simulink model "AN_Simulink_Model_v1"  (R2019b)
settings: Solver=VariableStepAuto  StartTime=0.0  StopTime=testtime  RelTol=1e-3
InitFcn:
  | AN_InitFcn_Callback
StopFcn:
  | AN_StopFcn_Callback
values from neighbouring files (symbols this model uses):
  alpha1 = 1.5e-6*100e3    (= 0.15)    [AN_Get_Model_Parameters.m]
  alpha2 = 1e-2*100e3    (= 1000)    [AN_Get_Model_Parameters.m]
  C1initphase = C1initphase + atan(CF/(-rzero))-atan((CF-pimag(2*i-1))/(-preal(2*i-1)))-atan((CF+pimag(2*i-1))/(-preal(2*i-1)))    [AN_Get_Model_Parameters.m]
  c1LPihc = ( Cihc - 2*pi*Fcihc ) / ( Cihc + 2*pi*Fcihc )    [AN_Get_Model_Parameters.m]
  c1LPohc = ( Cohc - 2*pi*Fcohc ) / ( Cohc + 2*pi*Fcohc )    [AN_Get_Model_Parameters.m]
  C1slope = 0.1    [AN_Get_Model_Parameters.m]
  c2LPihc = 2*pi*Fcihc / (2*pi*Fcihc + Cihc)    [AN_Get_Model_Parameters.m]
  c2LPohc = 2*pi*Fcohc / (2*pi*Fcohc + Cohc)    [AN_Get_Model_Parameters.m]
  C2slope = 0.2    [AN_Get_Model_Parameters.m]
  centerfreq = 165.4*(10^((bmplace+1.2)/(35/2.1)) - 1.0)    [AN_Get_Model_Parameters.m]
  CF = 2*pi*cf    [AN_Get_Model_Parameters.m]
  cf_factor = min(cfsat, 10^(cfslope*cf/1e3 + cfconst)) * 2.0    [AN_Get_Model_Parameters.m]
  cordiciterationswb = 52    [AN_Get_Model_Parameters.m]
  delta_phase = -2*pi*centerfreq*tdres    [AN_Get_Model_Parameters.m]
  fs_bilinear = 2*pi*cf/tan(2*pi*cf*tdres/2)    [AN_Get_Model_Parameters.m]
  gainihc = 1.0    (= 1)    [AN_Get_Model_Parameters.m]
  gainohc = 1.0    (= 1)    [AN_Get_Model_Parameters.m]
  ihcasym = 3.0    (= 3)    [AN_Get_Model_Parameters.m]
  m11 = 1/(C^2+5.9761e+003*C+2.5255e+007)    [AN_Get_Model_Parameters.m]
  m12 = -2*C^2+2*2.5255e+007    [AN_Get_Model_Parameters.m]
  m13 = C^2-5.9761e+003*C+2.5255e+007    [AN_Get_Model_Parameters.m]
  m14 = C^2+5.6665e+003*C    [AN_Get_Model_Parameters.m]
  m15 = -2*C^2    [AN_Get_Model_Parameters.m]
  m16 = C^2-5.6665e+003*C    [AN_Get_Model_Parameters.m]
  m21 = 1/(C^2+6.4255e+003*C+1.3975e+008)    [AN_Get_Model_Parameters.m]
  m22 = -2*C^2+2*1.3975e+008    [AN_Get_Model_Parameters.m]
  m23 = C^2-6.4255e+003*C+1.3975e+008    [AN_Get_Model_Parameters.m]
  m24 = C^2+5.8934e+003*C+1.7926e+008    [AN_Get_Model_Parameters.m]
  m25 = -2*C^2+2*1.7926e+008    [AN_Get_Model_Parameters.m]
  m26 = C^2-5.8934e+003*C+1.7926e+008    [AN_Get_Model_Parameters.m]
  m31 = 1/(C^2+2.4891e+004*C+1.2700e+009)    [AN_Get_Model_Parameters.m]
  m32 = -2*C^2+2*1.2700e+009    [AN_Get_Model_Parameters.m]
  m33 = C^2-2.4891e+004*C+1.2700e+009    [AN_Get_Model_Parameters.m]
  m34 = (3.1137e+003*C+6.9768e+008)    [AN_Get_Model_Parameters.m]
  m35 = 2*6.9768e+008    (= 1395360000)    [AN_Get_Model_Parameters.m]
  m36 = -3.1137e+003*C+6.9768e+008    [AN_Get_Model_Parameters.m]
  megainmax = 2    [AN_Get_Model_Parameters.m]
  minR = 0.05    [AN_Get_Model_Parameters.m]
  multFac = max(2.95*max(1.0,1.5-spont/100), 4.3-0.2*cf/1e3)    [AN_Get_Model_Parameters.m]
  norm_gainc1 = single(norm_gainc1)    [AN_Get_Model_Parameters.m]
  nSites = single(4)    [AN_Get_Model_Parameters.m]
  ohcasym = 7.0    (= 7)    [AN_Get_Model_Parameters.m]
  order_of_zero = half_order_pole    (= 5)    [AN_Get_Model_Parameters.m]
  pimag = zeros(11,1)    [AN_Get_Model_Parameters.m]
  preal = zeros(11,1)    [AN_Get_Model_Parameters.m]
  s0 = 12.0    (= 12)    [AN_Get_Model_Parameters.m]
  s1 = 5.0    (= 5)    [AN_Get_Model_Parameters.m]
  shift = 1.0/(1.0+ohcasym)    (= 0.125)    [AN_Get_Model_Parameters.m]
  spont = 100    [AN_Get_Model_Parameters.m]
  strength = (20.0e6)/(10^(corner/20))    (= 2000)    [AN_Get_Model_Parameters.m]
  tauwb = TauWBMax + (bmTaubm-bmTaumax)*(TauWBMax-TauWBMin)/(bmTaumax-bmTaumin)    [AN_Get_Model_Parameters.m]
  TauWBMax = Taumin + 0.2*(Taumax-Taumin)    [AN_Get_Model_Parameters.m]
  TauWBMin = TauWBMax/Taumax*Taumin    [AN_Get_Model_Parameters.m]
  wborder = 3    [AN_Get_Model_Parameters.m]
  x0 = s0*log((1.0/shift-1)/(1+exp(x1/s1)))    [AN_Get_Model_Parameters.m]
  x1 = 5.0    (= 5)    [AN_Get_Model_Parameters.m]
undefined symbols (not defined in the file or in its folder): bmTaumax, bmTaumin, cf, cihc, cohc, dfilt, Fs, jsin, norm_gainc2, tabs, tdres, trel, wbgain
libraries: dsparch4 x7, simulink x6, dspsrcs4 x3
(part 1 of 2)
settings Model: NumberOfSteps=50  Creator=mblun  LastModifiedBy=t96f346
settings OptimizationCC: BlockReduction=off  ConditionallyExecuteInputs=off  DefaultParameterBehavior=Inlined
settings DebuggingCC: UnderSpecifiedDimensionMsg=warning
settings SFSimCC: CustomCodeUndefinedFunction=UseInterfaceOnly

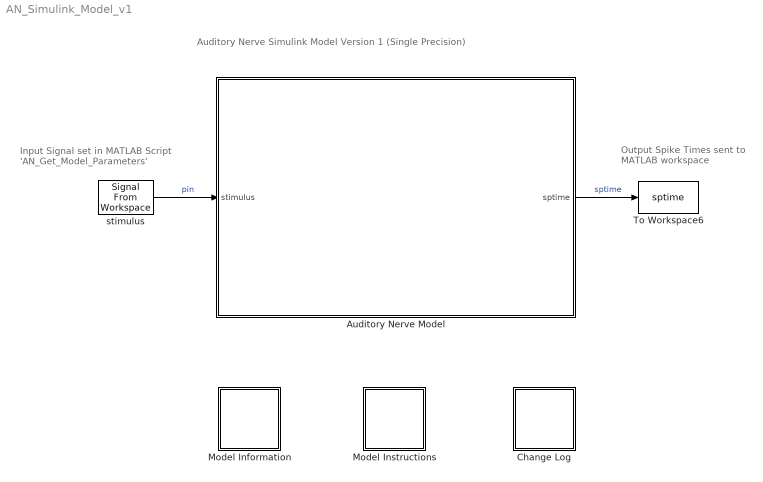
== system AN_Simulink_Model_v1 ==
  note: Input Signal set in MATLAB Script 'AN_Get_Model_Parameters'
  note: Auditory Nerve Simulink Model Version 1 (Single Precision)
  note: Output Spike Times sent to MATLAB workspace
  Auditory Nerve Model : Subsystem
  Change Log : Subsystem
  Model Information : Subsystem
  Model Instructions : Subsystem
  To Workspace6 : ToWorkspace  VariableName=sptime  SampleTime=-1
      settings: Save2DSignal=2-D array (concatenate along first dimension)
  "stimulus " : dspsrcs4/Signal From Workspace  X=RxSignal  Ts=tdres  nsamps=1  OutputAfterFinalValue=Setting to zero  ignoreOrWarnInputAndFrameLengths=off  OutputFrames=off
  wires:
  Auditory Nerve Model/1(sptime) -> To Workspace6/1  "sptime"
  "stimulus "/1 -> Auditory Nerve Model/1(stimulus)  "pin"

== system AN_Simulink_Model_v1/Auditory Nerve Model ==
  note: IHC
  note: OHC
  note: Input sound pressure waveform passes through middle ear filter
  note: Middle Ear output signal goes through broadly-tuned C2 filter and narrowly-tuned C1 filter in the model signal path
  note: C1/C2-filtered signals pass through the inner hair cell model (IHC), resulting in a relative transmembrane potential output
  note: Relative potential from IHC passes through the synapse model, which outputs the mean synaptic release rate of the neuron
  note: Mean synaptic release rate is input to the spike generator model, which uses a pseudo-random process to determine spike times for the neuron, along with various firing statistics of the neuron
  note: Middle Ear output signal goes through the gammatone filter of the control path. This is a feed-forward path which is used to tune the highly-sensitive C1 filter
  note: Gammatone filter output is passed to the outer-hearing cell model (OHC), which outputs a time constant to be used by the C1 filter
  note: The C1 filter time constant is input to a function which feeds an updated time-constant and associated gain back into the gammatone control path filter
  stimulus : Inport
  C1 Chirp Filter : Subsystem
  C2 Wideband Filter : Subsystem
  CP Wideband Gammatone Filter : Subsystem
  Middle Ear Filter : Subsystem
  Spike Generator : Subsystem
  Subsystem : Subsystem
  Subsystem1 : Subsystem
  Synapse Model : Subsystem
  f(tauc1) : Subsystem
  sptime : Outport  VectorParamsAs1DForOutWhenUnconnected=off
  wires:
  CP Wideband Gammatone Filter/1(output1) -> Subsystem1/1(wbout)  "wbout1"
  f(tauc1)/1(tauwb) -> CP Wideband Gammatone Filter/2(tauwb)  "tauwb"
  Subsystem1/1(tauc1) -> f(tauc1)/1(tauc1), C1 Chirp Filter/2(tauc1)  "tauc1"
  Middle Ear Filter/1(output) -> CP Wideband Gammatone Filter/3(stimulus), C1 Chirp Filter/1(meout), C2 Wideband Filter/1(stimulus)  "meout"
  stimulus/1 -> Middle Ear Filter/1(stimulus)  "pin"
  C1 Chirp Filter/1(output) -> Subsystem/2(C1filterout)  "C1filterout"
  Subsystem/1(ihcout) -> Synapse Model/1(ihcout)  "ihcout"
  C2 Wideband Filter/1(output) -> Subsystem/1(C2filterout)  "C2filterout"
  f(tauc1)/2(wbgain) -> CP Wideband Gammatone Filter/1(wbgain)  "wbgain"
  Synapse Model/1(synout) -> Spike Generator/1(synout)  "synout"
  Spike Generator/1(sptime) -> sptime/1  "sptime"

== system AN_Simulink_Model_v1/Change Log ==
  Change Log : simulink/Model-Wide Utilities/Model Info  Frame=on  DisplayStringWithTags=|  HorizontalTextAlignment=Left  LeftAlignmentValue=0.02
      | The following is the change log for the AN Simulink Model. Any major version changes should be 
      | documented and summarized below.
      | 
      | ------------------------------------------------------------------------------------------------------------------------------------
      | 
      | Version 1:
      | 	
      | 	- First Draft Version of Simulink Model by Matthew Blunt --- 08/07/2019
      | 
      | ------------------------------------------------------------------------------------------------------------------------------------
      | 
      | (Next Version Here)
      | 
      | 	- (Details and Changes Here)

== system AN_Simulink_Model_v1/Model Information ==
  "Model Information " : simulink/Model-Wide Utilities/Model Info  Frame=on  DisplayStringWithTags=|  HorizontalTextAlignment=Left  LeftAlignmentValue=0.02
      | Model Name: AN_Simulink_Model_v1
      | Created By: Matthew Blunt
      | Last Modification Date: 08/07/2019
      | Most Recently Modified By: Matthew Blunt
      | Model Version: 1
      | 
      | ------------------------------------------------------------------------------------------------------------------------------------
      | 
      | Description: This is a sample-based auditory nerve Simulink model, designed to closely replicate the 
      | auditory nerve model presented in the following publication:
      | 
      | 			Bruce, I.C., Erfani, Y., and Zilany, M.S.A. (2018). "A Phenomenological
      | 			model of the synapse between the inner hair cell and auditory nerve: 
      | 			Implications of limited neurotransmitter release sites," to appear in
      | 			Hearing Research. (Special Issue on "Computational Models in Hearing".)
      | 
      | It is important to also recognize the previous iterations of the phenomenological auditory 
      | nerve model, as they served as additional references during the design of the Simulink model.
      | 
      | ------------------------------------------------------------------------------------------------------------------------------------
      | 
      | This software was developed in conjunction with Flat Earth Inc
      | 
      | Copyright 2019 Flat Earth Inc
      | 
      | THE SOFTWARE IS PROVIDED "AS IS", WITHOUT WARRANTY OF ANY KIND, EXPRESS OR
      | IMPLIED, INCLUDING BUT NOT LIMITED TO THE WARRANTIES OF MERCHANTABILITY,
      | FITNESS FOR A PARTICULAR PURPOSE AND NONINFRINGEMENT. IN NO EVENT SHALL
      | THE AUTHORS OR COPYRIGHT HOLDERS BE LIABLE FOR ANY CLAIM, DAMAGES OR
      | OTHER LIABILITY, WHETHER IN AN ACTION OF CONTRACT, TORT OR OTHERWISE,
      | ARISING FROM, OUT OF OR IN CONNECTION WITH THE SOFTWARE OR THE USE OR
      | OTHER DEALINGS IN THE SOFTWARE.
      | 
      |    		Matthew Blunt
      |   		 Flat Earth Inc
      |    		985 Technology Blvd
      |    		Bozeman, MT 59718
      |    		support@flatearthinc.com

== system AN_Simulink_Model_v1/Model Instructions ==
  "Model Instructions " : simulink/Model-Wide Utilities/Model Info  Frame=on  DisplayStringWithTags=|  HorizontalTextAlignment=Left  LeftAlignmentValue=0.02
      | The following is a full set of instructions outlining the necessary steps to be taken in order to run the 
      | AN Simulink Model. Instructions can also be found in the readme file found in the
      | AN_Simulink_Model_v1_Doubles folder.
      | 
      | ------------------------------------------------------------------------------------------------------------------------------------
      | 
      | ** Quick Start Instructions **
      | 
      | If the user desires to simply run the model as is, refer to the Quick Start
      | Instructions pdf, which gives a quick visual tutorial on running the Auditory
      | Nerve Simulink Model.
      | 
      | ------------------------------------------------------------------------------------------------------------------------------------
      | 
      | ** Modify Model Instructions **
      | 
      | If the user desires to make modifications to the model before runtime,
      | refer to the Modify Model Instructions pdf, which gives a quick visual
      | tutorial on modifying the Auditory Nerve Simulink Model.
      | 
      | ------------------------------------------------------------------------------------------------------------------------------------
      | 
      | ** Verify Model Instructions **
      | 
      | If the user desires to verify model functionality against the original 
      | model source code, instructions are listed below, as well as in the readme.txt file
      | 
      | 1. Make sure MATLAB R2019a and a compatible C compiler are downloaded on the
      | machine the model will be running on. The C compiler is needed for C functions
      | used in the test/verification process. The compiler used for testing was the
      | MinGW-w64 C/C++ Compiler. This can be easily accessed for free in the Add-On
      | Explorer found in the MATLAB home tab.
      | 
      | 2. Open the AN_Simulink_Model_v1_Doubles folder in MATLAB. This is necessary in
      | order for the Simulink model to interact with MATLAB.
      | 
      | 3. Edit model parameters, if necessary. This can be done by adjusting the
      | overall model parameters set in the AN_Set_Model_Parameters script, or adjusting
      | other parameters in the AN_Get_Model_Parameters script. Both scripts are found
      | in the AN_Simulink_Model_v1_Doubles folder.
      | 
      | 4. Set the 'verificationflag' boolean to 'true' in the AN_Set_Model_Parameters
      | script. This enables the model to run the comparison C/MATLAB source functions
      | which are compared to the Simulink Model.
      | 
      | 5. Run the model. This is done by simply clicking the green 'Run' button
      | located at the top panel of Simulink. In addition, the model can be stepped
      | through in increments, using the 'Step Through' button to the right of the
      | 'Run' button.

== system AN_Simulink_Model_v1/Auditory Nerve Model/C1 Chirp Filter ==
  note: C1 Chirp Filter:
      |
      | Inputs : ME Filtered Signal (meout)
      | C1 Coefficients (a&b)
      | Normalizing Gain (norm_gain)
      |
      | Output : C1 Filtered Signal (c1filterout)
      |
      | - 10th Order IIR Bandpass Filter
      |
      | - Coefficients are determined in previous Get C1 Coefficients block
      |
      | - Implemented w/ Simulink biquad block
  note: Get C1 Coefficients
      |
      | Input : Pole-Shifting Feedback Parameter (rsigma)
      |
      | Outputs : C1 Coefficients (a&b)
      | Normalizing Gain (norm_gain)
      |
      | - Consists of various calculations to shift continuous-time pole locations according to rsigma feedback, then apply a bilinear transformation to bring the poles to the digital space before finding the coefficients for the C1 filter
  note: Calculate C1 Filter Output
      |
      | - Simply scale the output by cihc
  note: Calculate Pole-Shifting Parameter rsigma
      |
      | Input : C1 Feedback Time Constant (tauc1)
      |
      | Outputs : Pole-Shifting Parameter rsigma
      |
      | - Simple calculation to find rsigma from time constant feedback input
  meout : Inport
  tauc1 : Inport  Port=2
  C1 FIlter : Subsystem
  Calculate C1filterout : Subsystem
  Calculate rsigma : Subsystem
  Get C1 Coefficients : Subsystem
  To Workspace2 : ToWorkspace  VariableName=rsigma  SampleTime=-1
      settings: Save2DSignal=2-D array (concatenate along first dimension)
  output : Outport  VectorParamsAs1DForOutWhenUnconnected=off
  wires:
  meout/1 -> C1 FIlter/1(meout)
  C1 FIlter/1(Out1) -> Calculate C1filterout/1(C1filterouttmp)  "c1filterouttmp"
  Get C1 Coefficients/1(b0(5)) -> C1 FIlter/2(b0(5))
  Get C1 Coefficients/2(b0(3)) -> C1 FIlter/3(b0(3))
  Get C1 Coefficients/3(b0(1)) -> C1 FIlter/4(b0(1))
  Get C1 Coefficients/4(b1(5)) -> C1 FIlter/5(b1(5))
  Get C1 Coefficients/5(b1(3)) -> C1 FIlter/6(b1(3))
  Get C1 Coefficients/6(b1(1)) -> C1 FIlter/7(b1(1))
  Get C1 Coefficients/7(b2(5)) -> C1 FIlter/8(b2(5))
  Get C1 Coefficients/8(b2(3)) -> C1 FIlter/9(b2(3))
  Get C1 Coefficients/9(b2(1)) -> C1 FIlter/10(b2(1))
  Get C1 Coefficients/10(a2(5)) -> C1 FIlter/11(a2(5))
  Get C1 Coefficients/11(a2(3)) -> C1 FIlter/12(a2(3))
  Get C1 Coefficients/12(a2(1)) -> C1 FIlter/13(a2(1))
  Get C1 Coefficients/13(a1(1)) -> C1 FIlter/14(a1(1))
  Get C1 Coefficients/14(a1(3)) -> C1 FIlter/15(a1(3))
  Get C1 Coefficients/15(a1(5)) -> C1 FIlter/16(a1(5))
  Calculate C1filterout/1(C1filterout) -> output/1  "C1filterout"
  Calculate rsigma/1(rsigma) -> Get C1 Coefficients/1(rsigma), To Workspace2/1  "rsigma"
  tauc1/1 -> Calculate rsigma/1(tauc1)  "tauc1"

== system AN_Simulink_Model_v1/Auditory Nerve Model/C2 Wideband Filter ==
  note: C2 Wideband Filter:
      |
      | Input : ME Filtered Signal (meout)
      |
      | Output : C2 Filtered Signal (c2filterout)
      |
      | - 10th Order IIR Bandpass Filter
      |
      | - Coefficients are determined in AN_Get_Parameters init script
      |
      | - Implemented w/ Simulink biquad block
  note: Calculate C2 Filter Output:
      |
      | - Simply scale filter output
  stimulus : Inport
  Biquad Filter1 : dsparch4/Biquad Filter  FilterSource=Dialog parameters  CoeffSource=Specify via dialog  FilterObject=dfilt.df2tsos([1 0.3 0.4],[1 0.1 0.2])  IIRFiltStruct=Direct form II transposed  BiQuadCoeffs=C2coeffs  ScaleValues=1  IC=0  ICnum=0  ICden=0  a0Flag=Warning  optimizeScaleValues=on  ScaleValueMode=Specify via input port (g)  roundingMode=Floor  overflowMode=on  scaleValueFracLength=14  denProdOutputFracLength=30  denAccumFracLength=30  secondMemoryFracLength=15
      settings: SourceProductName=DSP System Toolbox
  Calculate C2filterout : Subsystem
  Gain : Gain  Gain=norm_gainc2/4
  output : Outport  VectorParamsAs1DForOutWhenUnconnected=off
  wires:
  stimulus/1 -> Biquad Filter1/1
  Biquad Filter1/1 -> Gain/1
  Gain/1 -> Calculate C2filterout/1(C2filterouttmp)  "c2filterouttmp"
  Calculate C2filterout/1(C2filterout) -> output/1  "C2filterout"

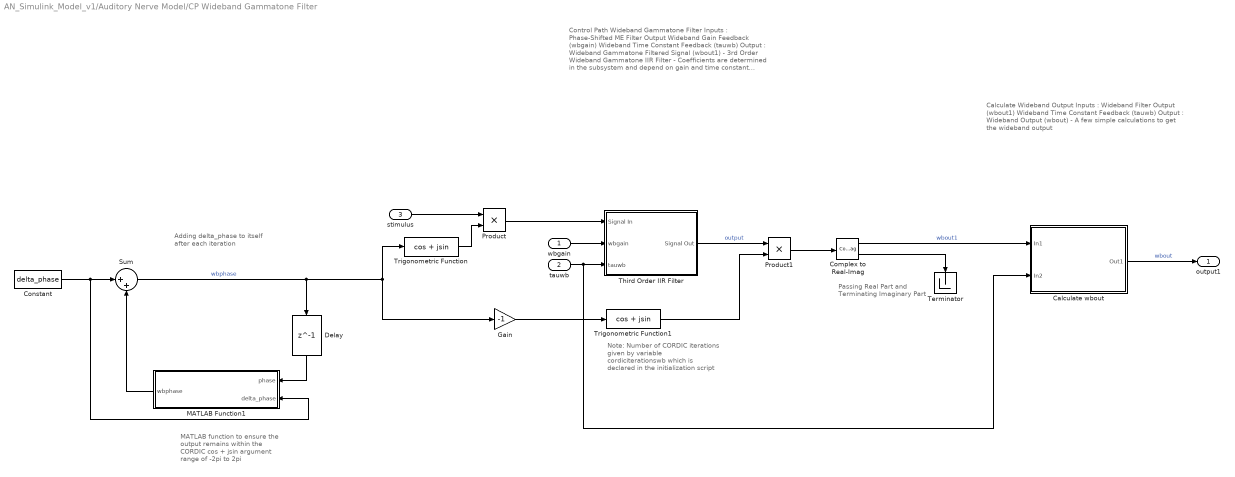
== system AN_Simulink_Model_v1/Auditory Nerve Model/CP Wideband Gammatone Filter ==
  note: Passing Real Part and Terminating Imaginary Part
  note: Note: Number of CORDIC iterations given by variable cordiciterationswb which is declared in the initialization script
  note: Adding delta_phase to itself after each iteration
  note: MATLAB function to ensure the output remains within the CORDIC cos + jsin argument range of -2pi to 2pi
  note: Control Path Wideband Gammatone Filter
      |
      | Inputs : Phase-Shifted ME Filter Output
      | Wideband Gain Feedback (wbgain)
      | Wideband Time Constant Feedback (tauwb)
      |
      | Output : Wideband Gammatone Filtered Signal (wbout1)
      |
      | - 3rd Order Wideband Gammatone IIR Filter
      |
      | - Coefficients are determined in the subsystem and depend on gain and time constant feedback
      |
      | - Implemented w/ Direct Form I Block Structure
  note: Calculate Wideband Output
      |
      | Inputs : Wideband Filter Output (wbout1)
      | Wideband Time Constant Feedback (tauwb)
      |
      | Output : Wideband Output (wbout)
      |
      | - A few simple calculations to get the wideband output
  wbgain : Inport
  tauwb : Inport  Port=2  OutDataTypeStr=single
  stimulus : Inport  Port=3  OutDataTypeStr=single
  Calculate wbout : Subsystem
  Complex to Real-Imag : ComplexToRealImag
  Constant : Constant  Value=delta_phase  OutDataTypeStr=single  SampleTime=-1
  Delay : Delay  DelayLength=1  InitialCondition=0  UseCircularBuffer=on
  Gain : Gain  Gain=-1  OutDataTypeStr=single
  MATLAB Function1 : MATLAB Function  TreatAsAtomicUnit=on
  Product : Product  OutDataTypeStr=single
  Product1 : Product  OutDataTypeStr=single
  Sum : Sum  Inputs=|++  OutDataTypeStr=single
  Terminator : Terminator
  Third Order IIR Filter : Subsystem
  Trigonometric Function : Trigonometry  Operator=cos + jsin  ApproximationMethod=CORDIC  NumberOfIterations=cordiciterationswb
  Trigonometric Function1 : Trigonometry  Operator=cos + jsin  ApproximationMethod=CORDIC  NumberOfIterations=cordiciterationswb
  output1 : Outport  VectorParamsAs1DForOutWhenUnconnected=off
  wires:
  Third Order IIR Filter/1(Signal Out) -> Product1/1  "output"
  Trigonometric Function/1 -> Product/2
  Constant/1 -> Sum/1, MATLAB Function1/2(delta_phase)
  stimulus/1 -> Product/1
  Product/1 -> Third Order IIR Filter/1(Signal In)
  Sum/1 -> Gain/1, Trigonometric Function/1, Delay/1  "wbphase"
  Product1/1 -> Complex to Real-Imag/1
  Complex to Real-Imag/1 -> Calculate wbout/1(In1)  "wbout1"
  Complex to Real-Imag/2 -> Terminator/1
  Gain/1 -> Trigonometric Function1/1
  Trigonometric Function1/1 -> Product1/2
  tauwb/1 -> Calculate wbout/2(In2), Third Order IIR Filter/3(tauwb)
  wbgain/1 -> Third Order IIR Filter/2(wbgain)
  Calculate wbout/1(Out1) -> output1/1  "wbout"
  Delay/1 -> MATLAB Function1/1(phase)
  MATLAB Function1/1(wbphase) -> Sum/2

== system AN_Simulink_Model_v1/Auditory Nerve Model/Middle Ear Filter ==
  note: Middle Ear Filter
      |
      | Input : Pressure Stimulus Waveform (pin or px)
      |
      | Output : Filtered Signal (meout)
      |
      | - 6th Order IIR Lowpass Filter
      |
      | - Coefficients are determined in AN_Get_Parameters init script
      |
      | - Implemented w/ Simulink biquad block
  stimulus : Inport
  Biquad Filter4 : dsparch4/Biquad Filter  FilterSource=Dialog parameters  CoeffSource=Specify via dialog  FilterObject=dfilt.df2tsos([1 0.3 0.4],[1 0.1 0.2])  IIRFiltStruct=Direct form II transposed  BiQuadCoeffs=[m14*m11 m15*m11 m16*m11 1 m12*m11 m13*m11; m24*m21 m25*m21 m26*m21 1 m22*m21 m23*m21; m34*m31 m35*m31 m36*m31 1 m32*m31 m33*m31]  ScaleValues=[1 1 1 1/megainmax]  IC=0  ICnum=0  ICden=0  a0Flag=Warning  optimizeScaleValues=on  ScaleValueMode=Specify via input port (g)  roundingMode=Floor  overflowMode=on  scaleValueFracLength=14  denProdOutputFracLength=30  denAccumFracLength=30  secondMemoryFracLength=15
      settings: SourceProductName=DSP System Toolbox
  To Workspace3 : ToWorkspace  VariableName=meout  SampleTime=-1
      settings: Save2DSignal=2-D array (concatenate along first dimension)
  output : Outport  VectorParamsAs1DForOutWhenUnconnected=off
  wires:
  stimulus/1 -> Biquad Filter4/1
  Biquad Filter4/1 -> To Workspace3/1, output/1  "output"

== system AN_Simulink_Model_v1/Auditory Nerve Model/Spike Generator ==
  note: 4-Site Synaptic Release & Adaptive Redocking
      |
      | Input : Synapse Output (synout) & Uniformly Distributed Random Number Vector between 0 and 1 (randNums)
      |
      | Output : Spike Times (sptime), Spike Count (spCount), Current Redocking Period (current_redocking_period), & Redocking Time Vector (trd_vector)
      |
      | - Implemented using Stateflow Chart and embedded MATLAB functions
      |
      | - Shows states of synaptic sites during simulation
  note: Calculation of Mean Spike Rate
      |
      | Input : Synapse Output (synout) & Redocking Time Vector (trd_vector)
      |
      | Output : Mean Spike Rate (meanrate)
      |
      | - Statistical Estimation of Mean Spike Rate to Account for Random Nature of Spike Generation Process
  synout : Inport
  Calculate Mean Spike Rate : Subsystem
  Random Number Generator : dspsrcs4/Signal From Workspace  X=randNums  Ts=1/Fs  nsamps=1  OutputAfterFinalValue=Setting to zero  ignoreOrWarnInputAndFrameLengths=off  OutputFrames=off
  Stateflow Logic Chart : Stateflow chart  BlockKeywords=__PRM__SERIALIZED__DATA__:Stateflow Chart,Stateflow Diagram  TreatAsAtomicUnit=on
  To Workspace1 : ToWorkspace  VariableName=meanrate  SampleTime=-1
      settings: Save2DSignal=2-D array (concatenate along first dimension)
  To Workspace2 : ToWorkspace  VariableName=trd_vector  SampleTime=-1
      settings: Save2DSignal=2-D array (concatenate along first dimension)
  To Workspace6 : ToWorkspace  VariableName=spCount  SampleTime=-1
      settings: Save2DSignal=2-D array (concatenate along first dimension)
  To Workspace7 : ToWorkspace  VariableName=current_redocking_period  SampleTime=-1
      settings: Save2DSignal=2-D array (concatenate along first dimension)
  sptime : Outport  VectorParamsAs1DForOutWhenUnconnected=off
  wires:
  Stateflow Logic Chart/3(current_redocking_period) -> To Workspace7/1
  Stateflow Logic Chart/4(trd_vector) -> Calculate Mean Spike Rate/2(trd_vector), To Workspace2/1  "trd_vector"
  Stateflow Logic Chart/1(sptime) -> sptime/1
  synout/1 -> Stateflow Logic Chart/1(synout), Calculate Mean Spike Rate/1(synout)  "synout"
  Stateflow Logic Chart/2(spCount) -> To Workspace6/1
  Random Number Generator/1 -> Stateflow Logic Chart/2(randNums)
  Calculate Mean Spike Rate/1(meanrate) -> To Workspace1/1  "meanrate"

== system AN_Simulink_Model_v1/Auditory Nerve Model/Subsystem ==
  note: Sum Nonlinear Function Outputs
  note: IHC C2 Nonlinear Logarithmic Transduction Function
      |
      | Input : C2 Filtered Signal (c2filterout)
      |
      | Output : C2 Transduction Function Output (c2vihctmp)
  note: IHC C1 Nonlinear Logarithmic Transduction Function
      |
      | Input : C1 Filtered Signal (c1filterout)
      |
      | Output : C1 Transduction Function Output (c1vihctmp)
  note: IHC Lowpass Filter
      |
      | Input : Sum of C1 and C2 Nonlinear Outputs (ihcnonlinout)
      |
      | Output : IHC Output (ihcout)
      |
      | - 7th Order IIR Lowpass Filter
      |
      | - Implemented using Simulink biquad
  C2filterout : Inport
  C1filterout : Inport  Port=2
  IHC C1 NL Logarithmic Function : Subsystem
  IHC C2 NL Logarithmic Function : Subsystem
  IHC LP Filter : Subsystem
  Sum1 : Sum  Inputs=|++
  To Workspace : ToWorkspace  VariableName=ihcout  SampleTime=-1
      settings: Save2DSignal=2-D array (concatenate along first dimension)
  ihcout : Outport  VectorParamsAs1DForOutWhenUnconnected=off
  wires:
  IHC C2 NL Logarithmic Function/1(output) -> Sum1/1  "c2vihctmp"
  IHC C1 NL Logarithmic Function/1(output) -> Sum1/2  "c1vihctmp"
  C1filterout/1 -> IHC C1 NL Logarithmic Function/1(stimulus)  "c1filterout"
  IHC LP Filter/1(output) -> To Workspace/1, ihcout/1  "ihcout"
  Sum1/1 -> IHC LP Filter/1(stimulus)  "ihcnonlinout"
  C2filterout/1 -> IHC C2 NL Logarithmic Function/1(stimulus)  "c2filterout"

== system AN_Simulink_Model_v1/Auditory Nerve Model/Subsystem1 ==
  note: OHC Lowpass Filter
      |
      | Inputs : OHC Nonlinear Output (ohcnonlinout)
      |
      | Output : LP Filtered OHC Output (ohcout)
      |
      | - 2nd Order IIR Lowpass Filter
      |
      | - Coefficients are determined in the init script
      |
      | - Implemented w/ Simulink biquad
  note: Nonlinear Function After OHC
      |
      | Input : LP Filtered OHC Output (ohcout)
      |
      | Output : Temporary C1 Time Constant (tmptauc1)
      |
      | - Nonlinear Function designed to convert the Lowpass Filter Output to a Time Varying Constant for the C1 Filter
  note: OHC Nonlinear Boltzman Function
      |
      | Input : Wideband Output (wbout)
      |
      | Output : OHC Nonlinear Output (ohcnonlinout)
      |
      | - 2nd Order Boltzman Function
  note: Calculate C1 Time Constant
      |
      | Input : Temporary C1 Time Constant (tmptauc1)
      |
      | Output : C1 Time Constant (tauc1)
      |
      | - A simple calculation to get the final C1 time constant value
  wbout : Inport
  Calculate tauc1 : Subsystem
  NL After OHC Function : Subsystem
  OHC LP Filter : Subsystem
  OHC NL Boltzman Function : Subsystem
  To Workspace1 : ToWorkspace  VariableName=tauc1  SampleTime=-1
      settings: Save2DSignal=2-D array (concatenate along first dimension)
  tauc1 : Outport  VectorParamsAs1DForOutWhenUnconnected=off
  wires:
  wbout/1 -> OHC NL Boltzman Function/1(stimulus)  "wbout"
  NL After OHC Function/1(output) -> Calculate tauc1/1(In1)  "tmptauc1"
  OHC LP Filter/1(output) -> NL After OHC Function/1(stimulus)  "ohcout"
  OHC NL Boltzman Function/1(output) -> OHC LP Filter/1(stimulus)  "ohcnonlinout"
  Calculate tauc1/1(Out1) -> To Workspace1/1, tauc1/1  "tauc1"

== system AN_Simulink_Model_v1/Auditory Nerve Model/Synapse Model ==
  note: NL Before PLA
      |
      | Input : IHC output (ihcout)
      |
      | Output : Power Law Adaptation Input (powerLawIn)
      |
      | - Adapted slightly from source code in order to avoid log10(0)
  ihcout : Inport
  NL Before PLA : Subsystem
  Power Law Adaptation : Subsystem
  synout : Outport  VectorParamsAs1DForOutWhenUnconnected=off
  wires:
  ihcout/1 -> NL Before PLA/1(ihcout)  "ihcout"
  NL Before PLA/1(powerLawIn) -> Power Law Adaptation/1(powerLawIn)  "powerLawIn"
  Power Law Adaptation/1(synout) -> synout/1  "synout"

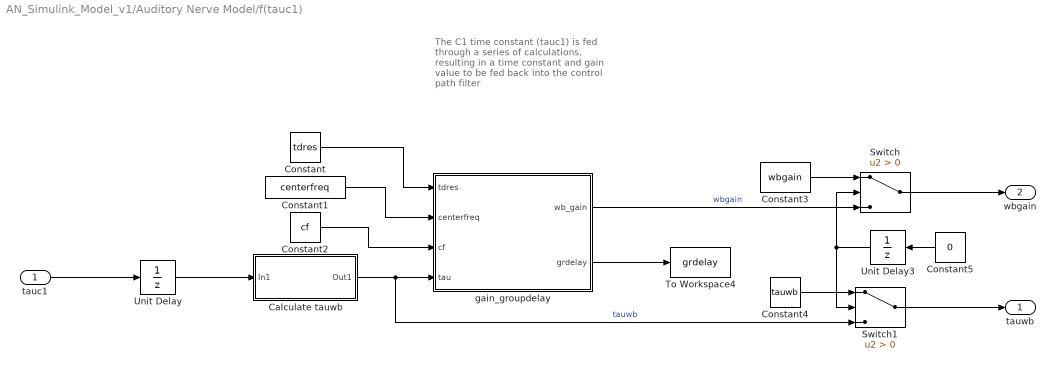
== system AN_Simulink_Model_v1/Auditory Nerve Model/f(tauc1) ==
  note: The C1 time constant (tauc1) is fed through a series of calculations, resulting in a time constant and gain value to be fed back into the control path filter
  tauc1 : Inport
  Calculate tauwb : Subsystem
  Constant : Constant  Value=tdres  OutDataTypeStr=single  SampleTime=-1
  Constant1 : Constant  Value=centerfreq  OutDataTypeStr=single  SampleTime=-1
  Constant2 : Constant  Value=cf  OutDataTypeStr=single  SampleTime=-1
  Constant3 : Constant  Value=wbgain  OutDataTypeStr=single  SampleTime=-1
  Constant4 : Constant  Value=tauwb  OutDataTypeStr=single  SampleTime=-1
  Constant5 : Constant  Value=0  OutDataTypeStr=single  SampleTime=-1
  Switch : Switch  Criteria=u2 > Threshold
  Switch1 : Switch  Criteria=u2 > Threshold
  To Workspace4 : ToWorkspace  VariableName=grdelay  SampleTime=-1
      settings: Save2DSignal=2-D array (concatenate along first dimension)
  Unit Delay : UnitDelay  SampleTime=-1  HasFrameUpgradeWarning=on
  Unit Delay3 : UnitDelay  InitialCondition=1  SampleTime=-1  HasFrameUpgradeWarning=on
  gain_groupdelay : MATLAB Function  TreatAsAtomicUnit=on
  tauwb : Outport  VectorParamsAs1DForOutWhenUnconnected=off
  wbgain : Outport  Port=2  VectorParamsAs1DForOutWhenUnconnected=off
  wires:
  Constant1/1 -> gain_groupdelay/2(centerfreq)
  tauc1/1 -> Unit Delay/1
  gain_groupdelay/1(wb_gain) -> Switch/3  "wbgain"
  Constant2/1 -> gain_groupdelay/3(cf)
  Constant/1 -> gain_groupdelay/1(tdres)
  Calculate tauwb/1(Out1) -> Switch1/3, gain_groupdelay/4(tau)  "tauwb"
  gain_groupdelay/2(grdelay) -> To Workspace4/1
  Switch/1 -> wbgain/1
  Unit Delay3/1 -> Switch/2, Switch1/2
  Switch1/1 -> tauwb/1
  Constant5/1 -> Unit Delay3/1
  Constant4/1 -> Switch1/1
  Constant3/1 -> Switch/1
  Unit Delay/1 -> Calculate tauwb/1(In1)

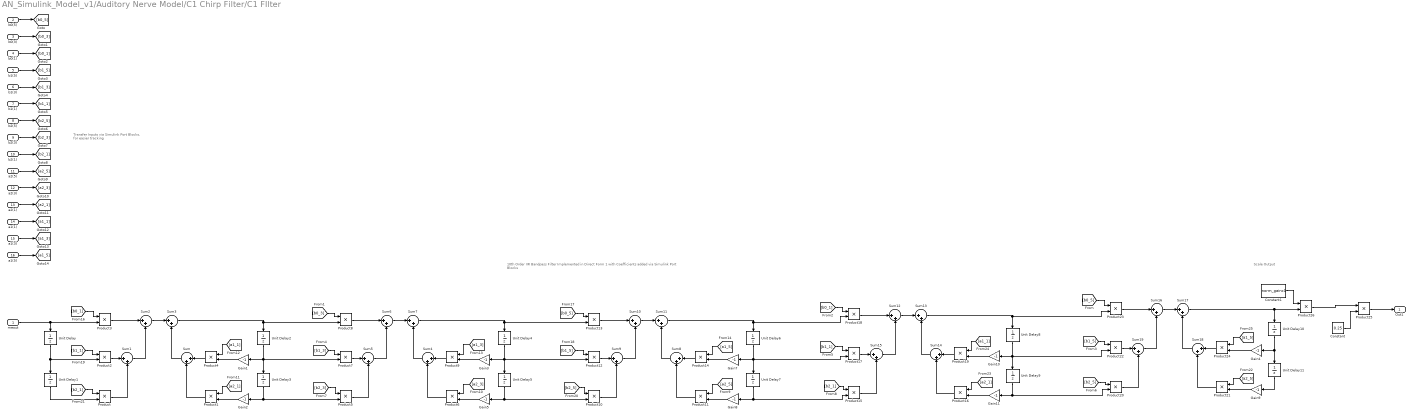
== system AN_Simulink_Model_v1/Auditory Nerve Model/C1 Chirp Filter/C1 FIlter ==
  note: Transfer Inputs via Simulink Port Blocks, for easier tracking
  note: 10th Order IIR Bandpass Filter Implemented in Direct Form 1 with Coefficients added via Simulink Port Blocks
  note: Scale Output
  meout : Inport
  b0(5) : Inport  Port=2
  b0(3) : Inport  Port=3
  b0(1) : Inport  Port=4
  b1(5) : Inport  Port=5
  b1(3) : Inport  Port=6
  b1(1) : Inport  Port=7
  b2(5) : Inport  Port=8
  b2(3) : Inport  Port=9
  b2(1) : Inport  Port=10
  a2(5) : Inport  Port=11
  a2(3) : Inport  Port=12
  a2(1) : Inport  Port=13
  a1(1) : Inport  Port=14
  a1(3) : Inport  Port=15
  a1(5) : Inport  Port=16
  Constant : Constant  Value=0.25  OutDataTypeStr=single  SampleTime=-1
  Constant1 : Constant  Value=norm_gainc1  OutDataTypeStr=single  SampleTime=-1
  Gain{1..5,7..11} (10 alike) : Gain  Gain=-1
  Product{,1..24} (25 alike) : Product
  Product25 : Product  OutDataTypeStr=single
  Product26 : Product  OutDataTypeStr=single
  Sum{,1..19} (20 alike) : Sum  Inputs=|++
  Unit Delay{,1..11} (12 alike) : UnitDelay  SampleTime=-1  HasFrameUpgradeWarning=on
  Out1 : Outport  VectorParamsAs1DForOutWhenUnconnected=off
  wires:
  [a1_5] -> Product14/1
  Product15/1 -> Sum15/2
  Product16/1 -> Sum14/2
  Sum5/1 -> Sum6/2
  Sum15/1 -> Sum12/2
  Unit Delay2/1 -> Product7/2, Unit Delay3/1, Gain1/1
  Unit Delay6/1 -> Product17/2, Unit Delay7/1, Gain7/1
  [b1_3] -> Product7/1
  Sum1/1 -> Sum2/2
  [b0_1] -> Product3/1
  Product4/1 -> Sum/1
  Unit Delay8/1 -> Product22/2, Unit Delay9/1, Gain10/1
  Product12/1 -> Sum9/1
  Sum17/1 -> Product26/2, Unit Delay10/1
  Product3/1 -> Sum2/1
  [b2_3] -> Product5/1
  Sum7/1 -> Product13/2, Unit Delay4/1
  [a2_1] -> Product1/1
  [b2_1] -> Product/1
  Product24/1 -> Sum18/1
  Unit Delay3/1 -> Product5/2, Gain2/1
  Product5/1 -> Sum5/2
  Unit Delay4/1 -> Product12/2, Unit Delay5/1, Gain3/1
  Sum13/1 -> Product23/2, Unit Delay8/1
  Sum3/1 -> Product8/2, Unit Delay2/1
  Sum4/1 -> Sum7/2
  Product19/1 -> Sum14/1
  Product7/1 -> Sum5/1
  Product10/1 -> Sum9/2
  Product20/1 -> Sum19/2
  [a1_5] -> Product24/1
  Sum6/1 -> Sum7/1
  [b0_5] -> Product13/1
  [a1_3] -> Product9/1
  Product22/1 -> Sum19/1
  Product8/1 -> Sum6/1
  meout/1 -> Product3/2, Unit Delay/1
  Product2/1 -> Sum1/1
  Sum11/1 -> Product18/2, Unit Delay6/1
  Unit Delay5/1 -> Product10/2, Gain5/1
  [b1_5] -> Product12/1
  Sum2/1 -> Sum3/1
  Product11/1 -> Sum8/2
  Sum19/1 -> Sum16/2
  [b2_5] -> Product20/1
  Product14/1 -> Sum8/1
  Product18/1 -> Sum12/1
  Sum8/1 -> Sum11/2
  [b0_3] -> Product8/1
  Sum12/1 -> Sum13/1
  [b0_5] -> Product23/1
  [b0_1] -> Product18/1
  [a1_1] -> Product19/1
  [a2_5] -> Product21/1
  Unit Delay/1 -> Unit Delay1/1, Product2/2
  Product17/1 -> Sum15/1
  Unit Delay7/1 -> Product15/2, Gain8/1
  Unit Delay10/1 -> Unit Delay11/1, Gain4/1
  [a2_5] -> Product11/1
  Unit Delay11/1 -> Gain9/1
  Product25/1 -> Out1/1
  Product23/1 -> Sum16/1
  Product9/1 -> Sum4/1
  [b1_1] -> Product17/1
  Product13/1 -> Sum10/1
  Product6/1 -> Sum4/2
  Sum9/1 -> Sum10/2
  Sum16/1 -> Sum17/1
  Product21/1 -> Sum18/2
  [b1_1] -> Product2/1
  Sum18/1 -> Sum17/2
  [b1_5] -> Product22/1
  [a2_1] -> Product16/1
  [a2_3] -> Product6/1
  Sum10/1 -> Sum11/1
  [b2_5] -> Product10/1
  [b2_1] -> Product15/1
  Product/1 -> Sum1/2
  Unit Delay9/1 -> Product20/2, Gain11/1
  Sum14/1 -> Sum13/2
  [a1_1] -> Product4/1
  Sum/1 -> Sum3/2
  Unit Delay1/1 -> Product/2
  Product1/1 -> Sum/2
  b0(5)/1 -> [b0_5]
  b0(3)/1 -> [b0_3]
  b0(1)/1 -> [b0_1]
  b1(5)/1 -> [b1_5]
  b1(3)/1 -> [b1_3]
  b1(1)/1 -> [b1_1]
  b2(5)/1 -> [b2_5]
  b2(3)/1 -> [b2_3]
  b2(1)/1 -> [b2_1]
  a2(5)/1 -> [a2_5]
  a2(3)/1 -> [a2_3]
  a2(1)/1 -> [a2_1]
  a1(1)/1 -> [a1_1]
  a1(3)/1 -> [a1_3]
  a1(5)/1 -> [a1_5]
  Gain1/1 -> Product4/2
  Gain2/1 -> Product1/2
  Gain3/1 -> Product9/2
  Gain5/1 -> Product6/2
  Gain7/1 -> Product14/2
  Gain8/1 -> Product11/2
  Gain10/1 -> Product19/2
  Gain11/1 -> Product16/2
  Gain4/1 -> Product24/2
  Gain9/1 -> Product21/2
  Constant/1 -> Product25/2
  Product26/1 -> Product25/1
  Constant1/1 -> Product26/1

== system AN_Simulink_Model_v1/Auditory Nerve Model/C1 Chirp Filter/Calculate C1filterout ==
  C1filterouttmp : Inport
  Gain1 : Gain  Gain=cihc
  C1filterout : Outport  VectorParamsAs1DForOutWhenUnconnected=off
  wires:
  C1filterouttmp/1 -> Gain1/1
  Gain1/1 -> C1filterout/1

== system AN_Simulink_Model_v1/Auditory Nerve Model/C1 Chirp Filter/Calculate rsigma ==
  note: Note: There are multiple HDL-friendly recipricol blocks. Use this block type for highest accuracy.
  note: Calculating rsigma using time constant feedback input
  tauc1 : Inport
  Constant2 : Constant  Value=bmTaumax  OutDataTypeStr=single  SampleTime=-1
  Reciprocal : Product  Inputs=/  SaturateOnIntegerOverflow=on  RndMeth=Zero
  Reciprocal1 : Product  Inputs=/  SaturateOnIntegerOverflow=on  RndMeth=Zero
  Subtract : Sum  Inputs=+-
  rsigma : Outport  VectorParamsAs1DForOutWhenUnconnected=off
  wires:
  tauc1/1 -> Reciprocal/1
  Constant2/1 -> Reciprocal1/1
  Reciprocal/1 -> Subtract/1
  Reciprocal1/1 -> Subtract/2
  Subtract/1 -> rsigma/1

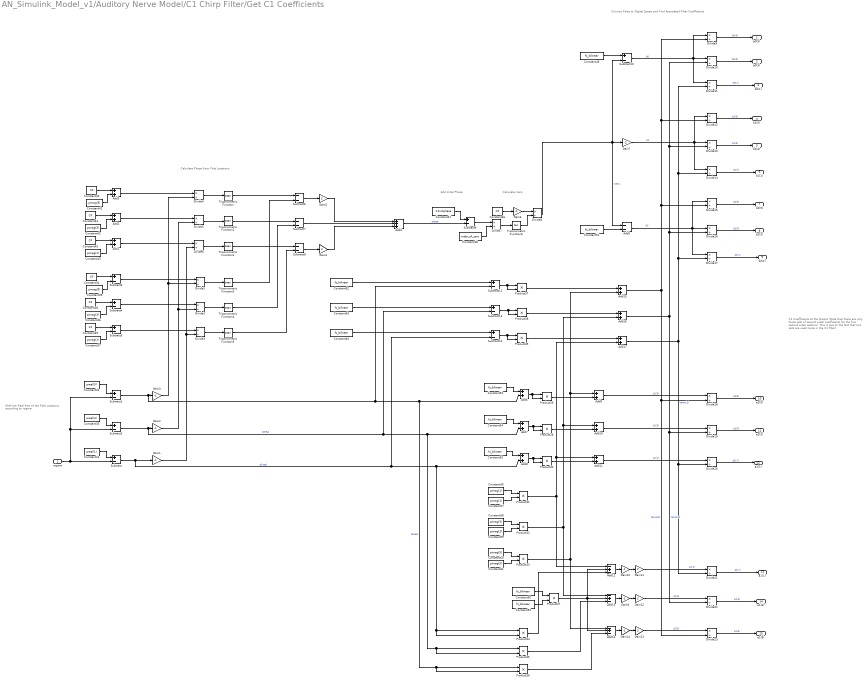
== system AN_Simulink_Model_v1/Auditory Nerve Model/C1 Chirp Filter/Get C1 Coefficients ==
  note: Calculate Phase from Pole Locations
  note: Shift the Real Part of the Pole Locations according to rsigma
  note: Add Initial Phase
  note: Calculate rzero
  note: Convert Poles to Digital Spcae and Find Associated Filter Coefficients
  note: C1 Coefficients at the Output (Note that there are only three sets of second order coefficients for the five second order sections. This is due to the fact that two sets are used twice in the C1 filter)
  rsigma : Inport
  Add{1..3,6..11,15..17} (12 alike) : Sum
  Add12 : Sum  Inputs=-+-
  Add13 : Sum  Inputs=-+-
  Add14 : Sum  Inputs=-+-
  Add4 : Sum  Inputs=+++
  Add5 : Sum  Inputs=--
  Constant31 : Constant  Value=preal(1)  OutDataTypeStr=single  SampleTime=-1
  Constant32 : Constant  Value=preal(5)  OutDataTypeStr=single  SampleTime=-1
  Constant33 : Constant  Value=preal(3)  OutDataTypeStr=single  SampleTime=-1
  Constant{34,38..40,44..46} (7 alike) : Constant  Value=CF  OutDataTypeStr=single  SampleTime=-1
  Constant{35,41,60..61} (4 alike) : Constant  Value=pimag(5)  OutDataTypeStr=single  SampleTime=-1
  Constant{36,42,58..59} (4 alike) : Constant  Value=pimag(3)  OutDataTypeStr=single  SampleTime=-1
  Constant{37,43,56..57} (4 alike) : Constant  Value=pimag(1)  OutDataTypeStr=single  SampleTime=-1
  Constant47 : Constant  Value=C1initphase  OutDataTypeStr=single  SampleTime=-1
  Constant48 : Constant  Value=order_of_zero  OutDataTypeStr=single  SampleTime=-1
  Constant{49..55,62..64} (10 alike) : Constant  Value=fs_bilinear  OutDataTypeStr=single  SampleTime=-1
  Divide{1..23} (23 alike) : Product  Inputs=*/  SaturateOnIntegerOverflow=on  RndMeth=Zero
  Gain{1..3,6,9..10,14} (7 alike) : Gain  Gain=-1
  Gain{4..5,11..13} (5 alike) : Gain  Gain=2
  Gain7 : Gain  Gain=-2
  Product{27..39} (13 alike) : Product
  Subtract{,1..5,9..13} (11 alike) : Sum  Inputs=+-
  Subtract6 : Sum  Inputs=--
  Subtract7 : Sum  Inputs=--
  Subtract8 : Sum  Inputs=--
  Trigonometric Function{,1..5} (6 alike) : Trigonometry  Operator=atan  ApproximationMethod=CORDIC
  Trigonometric Function6 : Trigonometry  Operator=tan  ApproximationMethod=CORDIC
  b0(5) : Outport  VectorParamsAs1DForOutWhenUnconnected=off
  b0(3) : Outport  Port=2  VectorParamsAs1DForOutWhenUnconnected=off
  b0(1) : Outport  Port=3  VectorParamsAs1DForOutWhenUnconnected=off
  b1(5) : Outport  Port=4  VectorParamsAs1DForOutWhenUnconnected=off
  b1(3) : Outport  Port=5  VectorParamsAs1DForOutWhenUnconnected=off
  b1(1) : Outport  Port=6  VectorParamsAs1DForOutWhenUnconnected=off
  b2(5) : Outport  Port=7  VectorParamsAs1DForOutWhenUnconnected=off
  b2(3) : Outport  Port=8  VectorParamsAs1DForOutWhenUnconnected=off
  b2(1) : Outport  Port=9  VectorParamsAs1DForOutWhenUnconnected=off
  a2(5) : Outport  Port=10  VectorParamsAs1DForOutWhenUnconnected=off
  a2(3) : Outport  Port=11  VectorParamsAs1DForOutWhenUnconnected=off
  a2(1) : Outport  Port=12  VectorParamsAs1DForOutWhenUnconnected=off
  a1(1) : Outport  Port=13  VectorParamsAs1DForOutWhenUnconnected=off
  a1(3) : Outport  Port=14  VectorParamsAs1DForOutWhenUnconnected=off
  a1(5) : Outport  Port=15  VectorParamsAs1DForOutWhenUnconnected=off
  wires:
  Add5/1 -> Divide17/1, Divide16/1, Divide15/1  "b2"
  Constant46/1 -> Gain6/1
  Divide6/1 -> Trigonometric Function2/1
  Divide18/1 -> a2(5)/1  "a2(5)"
  Subtract9/1 -> Divide7/1
  Constant33/1 -> Subtract2/1
  Add17/1 -> Divide21/2, Divide20/2, Divide17/2, Divide11/2, Divide14/2  "temp(1)"
  Product31/1 -> Add12/1, Add17/2, Add11/1
  Gain2/1 -> Divide5/2, Divide2/2
  Subtract8/1 -> Gain4/1
  rsigma/1 -> Subtract/2, Subtract1/2, Subtract2/2
  Gain1/1 -> Divide6/2, Divide3/2
  Add12/1 -> Gain10/1
  Constant52/1 -> Product27/2
  Add13/1 -> Gain9/1
  Add15/1 -> Divide23/2, Divide18/2, Divide9/2, Divide12/2, Divide15/2  "temp(5)"
  Add14/1 -> Gain14/1
  Product27/1 -> Add14/2, Add13/2, Add12/2
  Subtract2/1 -> Subtract12/2, Product35/2, Product35/1, Add7/2, Gain2/1  "p3real"
  Subtract1/1 -> Subtract11/2, Product36/2, Product36/1, Add6/2, Gain3/1  "p5real"
  Subtract/1 -> Subtract13/2, Product34/1, Product34/2, Add8/2, Gain1/1  "p1real"
  Divide5/1 -> Trigonometric Function1/1
  Constant59/1 -> Product32/2
  Add4/1 -> Subtract9/2  "phase"
  Product30/1 -> Add11/2
  Subtract13/1 -> Product39/2, Product39/1
  Product38/1 -> Add16/1
  Product39/1 -> Add17/1
  Divide21/1 -> a1(1)/1  "a1(1)"
  Product32/1 -> Add16/2, Add10/1, Add13/1
  Subtract7/1 -> Add4/2
  Constant62/1 -> Subtract11/1
  Constant58/1 -> Product32/1
  Divide2/1 -> Trigonometric Function4/1
  Subtract10/1 -> Divide11/1, Divide10/1, Divide9/1  "b0"
  Constant31/1 -> Subtract/1
  Trigonometric Function3/1 -> Subtract6/2
  Product36/1 -> Add14/3
  Add9/1 -> Divide18/1  "a2(5)"
  Product33/1 -> Add9/1, Add15/2, Add14/1
  Constant41/1 -> Add3/2
  Constant44/1 -> Add2/1
  Gain7/1 -> Divide14/1, Divide13/1, Divide12/1  "b1"
  Product35/1 -> Add13/3
  Add16/1 -> Divide22/2, Divide19/2, Divide10/2, Divide13/2, Divide16/2  "temp(3)"
  Constant63/1 -> Subtract12/1
  Divide8/1 -> Subtract10/2, Add5/1, Gain7/1  "rzero"
  Product34/1 -> Add12/3
  Trigonometric Function4/1 -> Subtract7/2
  Trigonometric Function5/1 -> Subtract8/2
  Subtract11/1 -> Product37/2, Product37/1
  Gain11/1 -> Divide21/1  "a1(1)"
  Gain12/1 -> Divide22/1  "a1(3)"
  Constant32/1 -> Subtract1/1
  Trigonometric Function6/1 -> Divide8/2
  Add8/1 -> Product30/2, Product30/1
  Constant40/1 -> Add3/1
  Gain6/1 -> Divide8/1
  Trigonometric Function1/1 -> Subtract7/1
  Add2/1 -> Divide5/1
  Subtract6/1 -> Gain5/1
  Gain13/1 -> Divide23/1  "a1(5)"
  Constant42/1 -> Add2/2
  Divide4/1 -> Trigonometric Function/1
  Product37/1 -> Add15/1
  Gain3/1 -> Divide4/2, Divide1/2
  Divide3/1 -> Trigonometric Function5/1
  Divide1/1 -> Trigonometric Function3/1
  Constant55/1 -> Add8/1
  Divide23/1 -> a1(5)/1  "a1(5)"
  Divide7/1 -> Trigonometric Function6/1
  Add6/1 -> Product29/2, Product29/1
  Product29/1 -> Add9/2
  Constant47/1 -> Subtract9/1
  Constant49/1 -> Subtract10/1
  Trigonometric Function2/1 -> Subtract8/1
  Subtract12/1 -> Product38/2, Product38/1
  Add3/1 -> Divide4/1
  Constant37/1 -> Subtract5/2
  Constant50/1 -> Product27/1
  Add11/1 -> Divide20/1  "a2(1)"
  Subtract5/1 -> Divide3/1
  Add1/1 -> Divide6/1
  Subtract4/1 -> Divide2/1
  Subtract3/1 -> Divide1/1
  Constant34/1 -> Subtract3/1
  Constant45/1 -> Add1/1
  Gain4/1 -> Add4/3
  Constant56/1 -> Product31/1
  Add7/1 -> Product28/2, Product28/1
  Gain5/1 -> Add4/1
  Constant51/1 -> Add5/2
  Product28/1 -> Add10/2
  Divide13/1 -> b1(3)/1  "b1(3)"
  Constant36/1 -> Subtract4/2
  Constant39/1 -> Subtract5/1
  Constant61/1 -> Product33/2
  Constant60/1 -> Product33/1
  Constant54/1 -> Add7/1
  Constant57/1 -> Product31/2
  Constant64/1 -> Subtract13/1
  Add10/1 -> Divide19/1  "a2(3)"
  Constant38/1 -> Subtract4/1
  Trigonometric Function/1 -> Subtract6/1
  Constant35/1 -> Subtract3/2
  Constant43/1 -> Add1/2
  Constant48/1 -> Divide7/2
  Constant53/1 -> Add6/1
  Divide17/1 -> b2(1)/1  "b2(1)"
  Divide12/1 -> b1(5)/1  "b1(5)"
  Divide20/1 -> a2(1)/1  "a2(1)"
  Divide11/1 -> b0(1)/1  "b0(1)"
  Divide14/1 -> b1(1)/1  "b1(1)"
  Divide15/1 -> b2(5)/1  "b2(5)"
  Divide10/1 -> b0(3)/1  "b0(3)"
  Divide22/1 -> a1(3)/1  "a1(3)"
  Divide9/1 -> b0(5)/1  "b0(5)"
  Divide19/1 -> a2(3)/1  "a2(3)"
  Divide16/1 -> b2(3)/1  "b2(3)"
  Gain10/1 -> Gain11/1
  Gain9/1 -> Gain12/1
  Gain14/1 -> Gain13/1

== system AN_Simulink_Model_v1/Auditory Nerve Model/C2 Wideband Filter/Calculate C2filterout ==
  C2filterouttmp : Inport
  Abs : Abs
  Constant : Constant  Value=cf  OutDataTypeStr=single  SampleTime=-1
  Constant1 : Constant  Value=10  OutDataTypeStr=single  SampleTime=-1
  Constant2 : Constant  Value=2e3  OutDataTypeStr=single  SampleTime=-1
  Constant3 : Constant  Value=cf  OutDataTypeStr=single  SampleTime=-1
  Divide : Product  Inputs=*/  SaturateOnIntegerOverflow=on  RndMeth=Zero
  Divide1 : Product  Inputs=*/  SaturateOnIntegerOverflow=on  RndMeth=Zero
  Product : Product
  Product1 : Product
  Product2 : Product
  C2filterout : Outport  VectorParamsAs1DForOutWhenUnconnected=off
  wires:
  C2filterouttmp/1 -> Product/1, Abs/1
  Abs/1 -> Product/2
  Product/1 -> Product1/1
  Constant/1 -> Product1/2
  Product1/1 -> Divide/1
  Constant1/1 -> Divide/2
  Product2/1 -> Divide1/1
  Constant2/1 -> Divide1/2
  Constant3/1 -> Product2/2
  Divide/1 -> Product2/1
  Divide1/1 -> C2filterout/1

== system AN_Simulink_Model_v1/Auditory Nerve Model/CP Wideband Gammatone Filter/Calculate wbout ==
  In1 : Inport
  In2 : Inport  Port=2
  Constant : Constant  Value=TauWBMax  OutDataTypeStr=single  SampleTime=-1
  Constant1 : Constant  Value=wborder  OutDataTypeStr=single  SampleTime=-1
  Constant2 : Constant  Value=cf  OutDataTypeStr=single  SampleTime=-1
  Constant3 : Constant  OutDataTypeStr=single  SampleTime=-1
  Constant4 : Constant  Value=5e3  OutDataTypeStr=single  SampleTime=-1
  Divide : Product  Inputs=*/  SaturateOnIntegerOverflow=on  RndMeth=Zero
  Divide1 : Product  Inputs=*/  SaturateOnIntegerOverflow=on  RndMeth=Zero
  Gain : Gain  Gain=10e3
  MinMax : MinMax  Function=max  Inputs=2
  Pow : Math  Operator=pow  RndMeth=Zero  SaturateOnIntegerOverflow=on
  Product : Product
  Product1 : Product
  Out1 : Outport  VectorParamsAs1DForOutWhenUnconnected=off
  wires:
  In2/1 -> Divide/1  "tauwb"
  In1/1 -> Product/1  "wbout1"
  Constant/1 -> Divide/2
  Divide/1 -> Pow/1
  Constant1/1 -> Pow/2
  Pow/1 -> Product/2
  Product/1 -> Gain/1
  Gain/1 -> Product1/1
  Divide1/1 -> MinMax/2
  Constant3/1 -> MinMax/1
  MinMax/1 -> Product1/2
  Product1/1 -> Out1/1
  Constant2/1 -> Divide1/1
  Constant4/1 -> Divide1/2

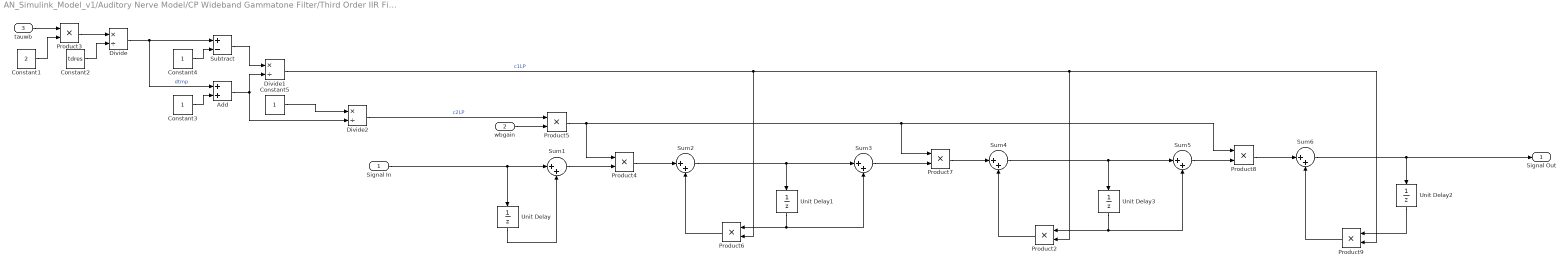
== system AN_Simulink_Model_v1/Auditory Nerve Model/CP Wideband Gammatone Filter/Third Order IIR Filter ==
  Signal In : Inport
  wbgain : Inport  Port=2
  tauwb : Inport  Port=3
  Add : Sum
  Constant1 : Constant  Value=2  OutDataTypeStr=single  SampleTime=-1
  Constant2 : Constant  Value=tdres  OutDataTypeStr=single  SampleTime=-1
  Constant3 : Constant  OutDataTypeStr=single  SampleTime=-1
  Constant4 : Constant  OutDataTypeStr=single  SampleTime=-1
  Constant5 : Constant  OutDataTypeStr=single  SampleTime=-1
  Divide : Product  Inputs=*/  SaturateOnIntegerOverflow=on  RndMeth=Zero
  Divide1 : Product  Inputs=*/  SaturateOnIntegerOverflow=on  RndMeth=Zero
  Divide2 : Product  Inputs=*/  SaturateOnIntegerOverflow=on  RndMeth=Zero
  Product{2..9} (8 alike) : Product
  Subtract : Sum  Inputs=+-
  Sum{1..6} (6 alike) : Sum  Inputs=|++
  Unit Delay{,1..3} (4 alike) : UnitDelay  SampleTime=-1  HasFrameUpgradeWarning=on
  Signal Out : Outport  VectorParamsAs1DForOutWhenUnconnected=off
  wires:
  Sum6/1 -> Signal Out/1, Unit Delay2/1
  Product8/1 -> Sum6/1
  Subtract/1 -> Divide1/1
  Product2/1 -> Sum4/2
  Signal In/1 -> Unit Delay/1, Sum1/1
  Product5/1 -> Product4/1, Product7/1, Product8/1
  Constant1/1 -> Product3/2
  Divide2/1 -> Product5/1  "c2LP"
  Unit Delay/1 -> Sum1/2
  Divide/1 -> Add/1, Subtract/1  "dtmp"
  Sum3/1 -> Product7/2
  Add/1 -> Divide2/2, Divide1/2
  Sum5/1 -> Product8/2
  Unit Delay1/1 -> Sum3/2, Product6/1
  Constant5/1 -> Divide2/1
  Product7/1 -> Sum4/1
  Product9/1 -> Sum6/2
  Unit Delay3/1 -> Sum5/2, Product2/1
  Sum2/1 -> Sum3/1, Unit Delay1/1
  Product6/1 -> Sum2/2
  Sum4/1 -> Sum5/1, Unit Delay3/1
  tauwb/1 -> Product3/1
  Product3/1 -> Divide/1
  Constant4/1 -> Subtract/2
  wbgain/1 -> Product5/2
  Unit Delay2/1 -> Product9/1
  Product4/1 -> Sum2/1
  Constant2/1 -> Divide/2
  Sum1/1 -> Product4/2
  Constant3/1 -> Add/2
  Divide1/1 -> Product6/2, Product9/2, Product2/2  "c1LP"

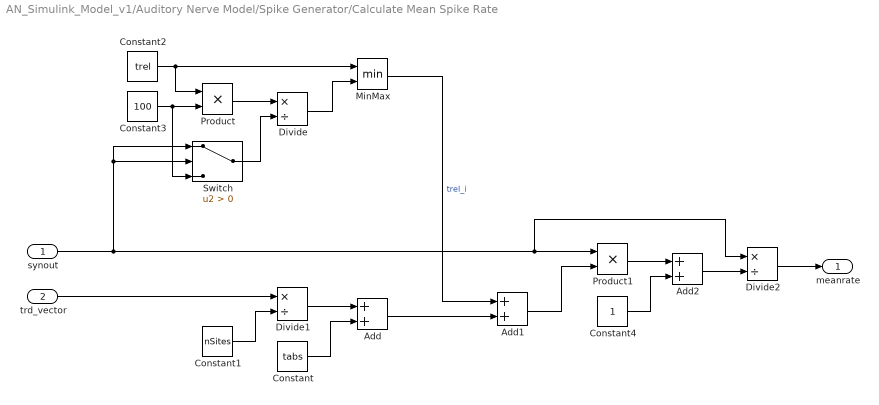
== system AN_Simulink_Model_v1/Auditory Nerve Model/Spike Generator/Calculate Mean Spike Rate ==
  synout : Inport
  trd_vector : Inport  Port=2
  Add : Sum
  Add1 : Sum
  Add2 : Sum
  Constant : Constant  Value=tabs  SampleTime=-1
  Constant1 : Constant  Value=nSites  SampleTime=-1
  Constant2 : Constant  Value=trel  SampleTime=-1
  Constant3 : Constant  Value=100  SampleTime=-1
  Constant4 : Constant  SampleTime=-1
  Divide : Product  Inputs=*/  SaturateOnIntegerOverflow=on  RndMeth=Zero
  Divide1 : Product  Inputs=*/  SaturateOnIntegerOverflow=on  RndMeth=Zero
  Divide2 : Product  Inputs=*/  SaturateOnIntegerOverflow=on  RndMeth=Zero
  MinMax : MinMax  Inputs=2
  Product : Product
  Product1 : Product
  Switch : Switch  Criteria=u2 > Threshold
  meanrate : Outport  VectorParamsAs1DForOutWhenUnconnected=off
  wires:
  synout/1 -> Switch/1, Switch/2, Divide2/1, Product1/1
  trd_vector/1 -> Divide1/1
  Constant2/1 -> MinMax/1, Product/1
  Constant3/1 -> Switch/3, Product/2
  Product/1 -> Divide/1
  Divide/1 -> MinMax/2
  MinMax/1 -> Add1/1  "trel_i"
  Constant1/1 -> Divide1/2
  Divide1/1 -> Add/1
  Constant/1 -> Add/2
  Add/1 -> Add1/2
  Constant4/1 -> Add2/2
  Add1/1 -> Product1/2
  Product1/1 -> Add2/1
  Add2/1 -> Divide2/2
  Divide2/1 -> meanrate/1
  Switch/1 -> Divide/2

== system AN_Simulink_Model_v1/Auditory Nerve Model/Subsystem/IHC C1 NL Logarithmic Function ==
  note: Nonlinear log
  stimulus : Inport
  Abs : Abs
  Add2 : Sum
  Compare To Zero : simulink/Logic and Bit Operations/Compare To Zero  relop=<  OutDataTypeStr=boolean
  Constant10 : Constant  Value=strength  OutDataTypeStr=single  SampleTime=-1
  Constant11 : Constant  OutDataTypeStr=single  SampleTime=-1
  Constant12 : Constant  Value=C1slope  OutDataTypeStr=single  SampleTime=-1
  Log : Math  Operator=log  SaturateOnIntegerOverflow=on
  Product1 : Product
  Product2 : Product
  Subsystem : Subsystem
  Switch : Switch  Criteria=u2 > Threshold
  output : Outport  VectorParamsAs1DForOutWhenUnconnected=off
  wires:
  stimulus/1 -> Subsystem/1(x), Compare To Zero/1, Abs/1  "x"
  Abs/1 -> Product1/1
  Constant10/1 -> Product1/2
  Constant11/1 -> Add2/2
  Product1/1 -> Add2/1
  Add2/1 -> Log/1
  Log/1 -> Product2/1
  Constant12/1 -> Product2/2
  Product2/1 -> Switch/3, Subsystem/2(In2)
  Compare To Zero/1 -> Subsystem/Enable, Switch/2
  Subsystem/1(Out1) -> Switch/1
  Switch/1 -> output/1

== system AN_Simulink_Model_v1/Auditory Nerve Model/Subsystem/IHC C2 NL Logarithmic Function ==
  note: Nonlinear log
  stimulus : Inport
  Abs : Abs
  Add2 : Sum
  Compare To Zero : simulink/Logic and Bit Operations/Compare To Zero  relop=<  OutDataTypeStr=boolean
  Constant10 : Constant  Value=strength  OutDataTypeStr=single  SampleTime=-1
  Constant11 : Constant  OutDataTypeStr=single  SampleTime=-1
  Constant12 : Constant  Value=C2slope  OutDataTypeStr=single  SampleTime=-1
  Gain : Gain  Gain=-1
  Log : Math  Operator=log  SaturateOnIntegerOverflow=on
  Product1 : Product
  Product2 : Product
  Subsystem : Subsystem
  Switch : Switch  Criteria=u2 > Threshold  OutDataTypeStr=single
  output : Outport  VectorParamsAs1DForOutWhenUnconnected=off
  wires:
  stimulus/1 -> Subsystem/2(In1), Compare To Zero/1, Abs/1  "x"
  Abs/1 -> Product1/1
  Constant10/1 -> Product1/2
  Constant11/1 -> Add2/2
  Product1/1 -> Add2/1
  Add2/1 -> Log/1
  Log/1 -> Product2/1
  Constant12/1 -> Product2/2
  Gain/1 -> output/1  "C2vihctmp"
  Compare To Zero/1 -> Switch/2, Subsystem/Enable
  Product2/1 -> Switch/3, Subsystem/1(In2)  "xx"
  Switch/1 -> Gain/1
  Subsystem/1(Out1) -> Switch/1
